simulink model "chap5_eye_hw3"  (R2017a)
settings: Solver=ode45  StartTime=0.0  StopTime=1.0  FixedStep=.0001  MaxStep=.002  RelTol=1e-3  EnableMultiTasking=on
settings Model: Creator=wintersj  LastModifiedBy=wintersj
settings DataIOCC: LimitDataPoints=on  SaveFormat=Array  SignalLoggingSaveFormat=ModelDataLogs
settings OptimizationCC: ExpressionDepthLimit=2147483647  LifeSpan=inf
settings DebuggingCC: UnderspecifiedInitializationDetection=Classic  MergeDetectMultiDrivingBlocksExec=none  MaxConsecutiveZCsMsg=none  SolverPrmCheckMsg=warning  FcnCallInpInsideContextMsg=warning  StateNameClashWarn=warning  SFUnexpectedBacktrackingDiag=warning  SFNoUnconditionalDefaultTransitionDiag=warning  SFExecutionAtInitializationDiag=none
settings HardwareCC: ProdBitPerPointer=32  ProdBitPerSizeT=32  ProdBitPerPtrDiffT=32  ProdLargestAtomicFloat=None  ProdIntDivRoundTo=Undefined  ProdEndianess=Unspecified  ProdWordSize=32  ProdHWDeviceType=32-bit Generic
settings ModelReferenceCC: PropagateSignalLabelsOutOfModel=off
settings GRTTargetCC: TargetLangStandard=C89/C90 (ANSI)  GeneratePreprocessorConditionals=Disable all  CombineOutputUpdateFcns=off  GRTInterface=on
settings ConfigComp: CovMetricSettings=dw  CovHtmlReporting=on  CovSaveCumulativeToWorkspaceVar=on  CovSaveSingleToWorkspaceVar=on  CovExternalEMLEnable=off

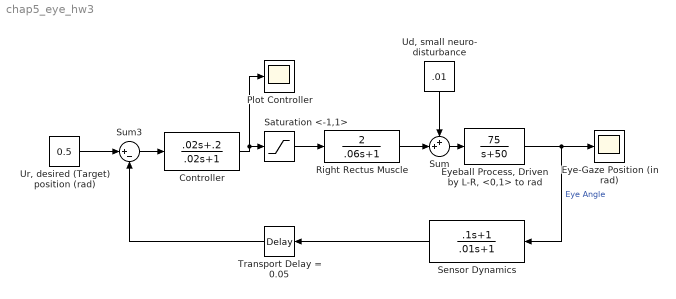
== system chap5_eye_hw3 ==
  Controller : TransferFcn  Numerator=[.02 .2]  Denominator=[.02 1]
  Eye-Gaze Position (in rad) : Scope
  "Eyeball Process, Driven by L-R, <0,1> to rad" : TransferFcn  Numerator=[75]  Denominator=[1 50]
  "Plot Controller " : Scope
  Right Rectus Muscle : TransferFcn  Numerator=[2]  Denominator=[.06 1]
  Saturation <-1,1> : Saturate  UpperLimit=1  LowerLimit=-1
  Sensor Dynamics : TransferFcn  Numerator=[.1 1]  Denominator=[.01 1]
  Sum : Sum  Inputs=++|
  Sum3 : Sum  Inputs=|+-
  Transport Delay = 0.05 : TransportDelay  DelayTime=.05
  "Ud, small neuro- disturbance" : Constant  Value=.01
  "Ur, desired (Target) position (rad)" : Constant  Value=0.5
  wires:
  Sum/1 -> "Eyeball Process, Driven by L-R, <0,1> to rad"/1
  "Eyeball Process, Driven by L-R, <0,1> to rad"/1 -> Eye-Gaze Position (in rad)/1, Sensor Dynamics/1  "Eye Angle"
  "Ud, small neuro- disturbance"/1 -> Sum/1
  Sensor Dynamics/1 -> Transport Delay = 0.05/1
  Transport Delay = 0.05/1 -> Sum3/2
  "Ur, desired (Target) position (rad)"/1 -> Sum3/1
  Right Rectus Muscle/1 -> Sum/2
  Sum3/1 -> Controller/1
  Controller/1 -> "Plot Controller "/1, Saturation <-1,1>/1
  Saturation <-1,1>/1 -> Right Rectus Muscle/1
